simulink model "exp5_7_2"  (Simulink 6.6)
settings: Solver=ode45  StartTime=0.0  StopTime=10.0  RelTol=1e-3
settings Model: Creator=Administrator  LastModifiedBy=Administrator  ExtModeTrigMode=oneshot  ExtModeArmWhenConnect=off
settings DataIOCC: LimitDataPoints=off
settings OptimizationCC: BlockReduction=off  BooleanDataType=off
settings DebuggingCC: SignalResolutionControl=TryResolveAllWithWarning  SolverPrmCheckMsg=none  MultiTaskDSMMsg=warning  MultiTaskCondExecSysMsg=none  StrictBusMsg=None
settings HardwareCC: TargetUnknown=on
settings RTWCC: IncludeERTFirstTime=on

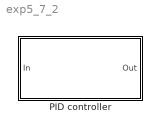
== system exp5_7_2 ==
  PID controller : Subsystem  mask(PID controller){kp=2, ki=3, kd=10}
      mask prompts: kp "the parameter of P"; ki "the parameter of I"; kd "the parameter of D"
      mask help: please set the parameters of PID, this is modified by Wang Xiaoping.
      mask Help:
      | This block implements a PID controller where parameters are
      | entered for the Proportional,Integral and Derivative terms.
      mask Display: disp('PID')

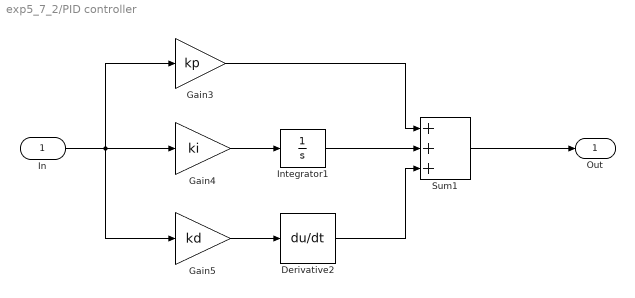
== system exp5_7_2/PID controller ==
  In : Inport
  Derivative2 : Derivative
  Gain3 : Gain  Gain=kp  SaturateOnIntegerOverflow=on
  Gain4 : Gain  Gain=ki  SaturateOnIntegerOverflow=on
  Gain5 : Gain  Gain=kd  SaturateOnIntegerOverflow=on
  Integrator1 : Integrator
  Sum1 : Sum  Inputs=+++  SaturateOnIntegerOverflow=on  InputSameDT=on
  Out : Outport
  wires:
  Gain4/1 -> Integrator1/1
  Gain5/1 -> Derivative2/1
  Gain3/1 -> Sum1/1
  Integrator1/1 -> Sum1/2
  Derivative2/1 -> Sum1/3
  Sum1/1 -> Out/1
  In/1 -> Gain4/1, Gain3/1, Gain5/1
